simulink model "Linearity in Parameter"  (R2015a)
settings: Solver=ode45  StartTime=0.0  StopTime=10  RelTol=1e-3
settings Model: Creator=ominub  LastModifiedBy=ominub

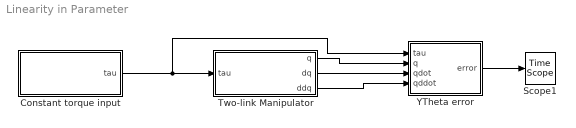
== system Linearity in Parameter ==
  Constant torque input : Subsystem
  Scope1 : TimeScope
  Two-link Manipulator : Subsystem
  YTheta error : MATLAB Function  TreatAsAtomicUnit=on
  wires:
  Constant torque input/1(tau) -> YTheta error/1(tau), Two-link Manipulator/1(tau)
  Two-link Manipulator/2(dq) -> YTheta error/3(qdot)
  Two-link Manipulator/3(ddq) -> YTheta error/4(qddot)
  Two-link Manipulator/1(q) -> YTheta error/2(q)
  YTheta error/1(error) -> Scope1/1

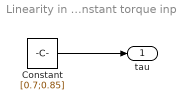
== system Linearity in Parameter/Constant torque input ==
  Constant : Constant  Value=[0.7;0.85]
  tau : Outport
  wires:
  Constant/1 -> tau/1

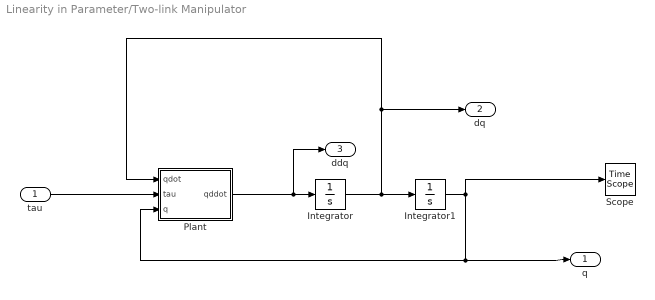
== system Linearity in Parameter/Two-link Manipulator ==
  tau : Inport
  Integrator : Integrator  InitialCondition=[0 0]
  Integrator1 : Integrator  InitialCondition=[0 0]
  Plant : MATLAB Function  TreatAsAtomicUnit=on
  Scope : TimeScope
  q : Outport
  dq : Outport  Port=2
  ddq : Outport  Port=3
  wires:
  Plant/1(qddot) -> ddq/1, Integrator/1
  Integrator/1 -> dq/1, Plant/1(qdot), Integrator1/1
  Integrator1/1 -> q/1, Plant/3(q), Scope/1
  tau/1 -> Plant/2(tau)

== matlab function Linearity in Parameter/Two-link Manipulator/Plant ==
  data: qdot input; tau input; qddot output; q input
function qddot = fcn(qdot,tau,q)
%#codegen
M1=1;
M2=0.8;
I1=0.05;
I2=0.03;
L1=1.2;
L2=0.8;
Lc1=L1/2;
Lc2=L2/2;
g=9.8;

D=[M1*Lc1^2+M2*(L1^2+Lc2^2+2*L1*Lc2*cos(q(2)))+I1+I2 , M2*(Lc2^2+L1*Lc2*cos(q(2)))+I2 ;...
   M2*(Lc2^2+L1*Lc2*cos(q(2)))+I2                    , M2*Lc2^2+I2];
C=[-(M2*L1*Lc2*sin(q(2)))*qdot(2) , -(M2*L1*Lc2*sin(q(2)))*(qdot(1)+qdot(2));...
    (M2*L1*Lc2*sin(q(2)))*qdot(1) , 0];
G=[(M1*Lc1+M2*L1)*g*cos(q(1))+M2*Lc2*g*cos(q(1)+q(2)) ; M2*Lc2*g*cos(q(1)+q(2))];

qddot=inv(D)*(tau-C*qdot-G);

== matlab function Linearity in Parameter/YTheta error ==
  data: tau input; q input; qdot input; qddot input; error output
function error = fcn(tau,q,qdot,qddot)
%#codegen
M1=1;
M2=0.8;
I1=0.05;
I2=0.03;
L1=1.2;
L2=0.8;
Lc1=L1/2;
Lc2=L2/2;
g=9.8;
Y=[qddot(1) , cos(q(2))*(2*qddot(1)+qddot(2))-sin(q(2))*(qdot(2)^2+2*qdot(1)*qdot(2)) , qddot(2)          , g*cos(q(1)) , g*cos(q(1)+q(2)) ;...
    0       , cos(q(2))*qddot(1)+sin(q(2))*qdot(1)^2                                  , qddot(1)+qddot(2) ,  0          , g*cos(q(1)+q(2)) ];
Theta=[M1*Lc1^2+M2*(L1^2+Lc2^2)+I1+I2;M2*L1*Lc2;M2*Lc2^2+I2;M1*Lc1+M2*L1;M2*Lc2];
    error=tau-Y*Theta;
